simulink model "FWLowModel"  (R2020b)
settings: Solver=VariableStepAuto  StartTime=0.0  StopTime=inf  RelTol=1e-3
libraries: uavalgslib x1
settings Model: EnablePacing=on  Creator=ISR  LastModifiedBy=chenjiaqing

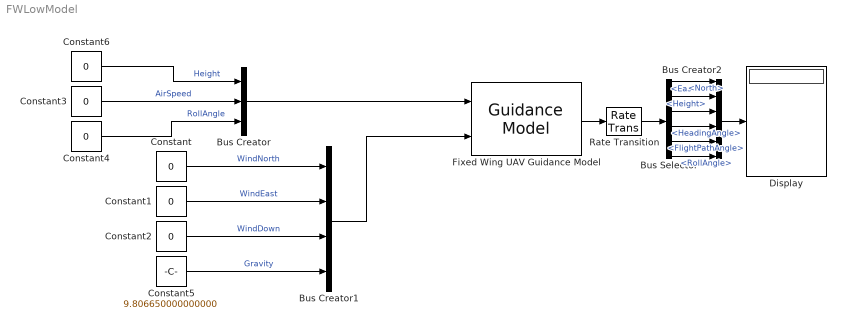
== system FWLowModel ==
  Bus Creator : BusCreator  Inputs=3  OutDataTypeStr=Bus: FixedWingControlBus  NonVirtualBus=on
  Bus Creator1 : BusCreator  Inputs=4  OutDataTypeStr=Bus: FixedWingEnvironmentBus  NonVirtualBus=on
  Bus Creator2 : BusCreator  Inputs=6
  Bus Selector : BusSelector  OutputSignals=North,East,Height,HeadingAngle,FlightPathAngle,RollAngle
  Constant{,1..4,6} (6 alike) : Constant  Value=0
  Constant5 : Constant  Value=9.806650000000000
  Display : Display
  Fixed Wing UAV Guidance Model : uavalgslib/Guidance Model  ModelType=FixedWingGuidance  SpecifiedDataType=double  SimulateUsing=Code generation  InitialWorldPositionMultirotor=[0; 0; 0]  InitialWorldVelocityMultirotor=[0; 0; 0]  InitialEulerZYXMultirotor=[0; 0; 0]  InitialBodyAngularRateRPYMultirotor=[0; 0; 0]  InitialThrustMultirotor=0  InitialNorthFixedWing=0  InitialEastFixedWing=0  InitialHeightFixedWing=0  InitialAirSpeedFixedWing=0  InitialHeadingAngleFixedWing=0  InitialFlightPathAngleFixedWing=0  InitialRollAngleFixedWing=0  InitialRollAngleRateFixedWing=0  PDRollMultirotor=[3402.97,116.67]  PDPitchMultirotor=[3402.97, 116.67]  PYawRateMultirotor=1950  PThrustMultirotor=3900  MassMultirotor=0.1  PHeightFixedWing=0.78  PHeadingAngleFixedWing=3.9  PFlightPathAngleFixedWing=3.9  PDRollFixedWing="[5.4448      4.6668]"  PAirSpeedFixedWing=7.8  FlightPathAngleLimitsFixedWing=[-pi/4, pi/4]  StateBusName='FixedWingStateBus'  ControlBusName='FixedWingControlBus'  EnvironmentBusName='FixedWingEnvironmentBus'  DataType=double
      settings: SourceProductName=UAV Toolbox
  Rate Transition : RateTransition  OutPortSampleTime=0.1
  wires:
  Fixed Wing UAV Guidance Model/1 -> Rate Transition/1
  Bus Selector/4 -> Bus Creator2/4  "<HeadingAngle>"
  Bus Creator2/1 -> Display/1
  Bus Selector/5 -> Bus Creator2/5  "<FlightPathAngle>"
  Bus Selector/6 -> Bus Creator2/6  "<RollAngle>"
  Bus Selector/2 -> Bus Creator2/2  "<East>"
  Bus Selector/3 -> Bus Creator2/3  "<Height>"
  Rate Transition/1 -> Bus Selector/1
  Constant3/1 -> Bus Creator/2  "AirSpeed"
  Constant4/1 -> Bus Creator/3  "RollAngle"
  Bus Selector/1 -> Bus Creator2/1  "<North>"
  Constant2/1 -> Bus Creator1/3  "WindDown"
  Bus Creator/1 -> Fixed Wing UAV Guidance Model/1
  Constant/1 -> Bus Creator1/1  "WindNorth"
  Constant1/1 -> Bus Creator1/2  "WindEast"
  Bus Creator1/1 -> Fixed Wing UAV Guidance Model/2
  Constant6/1 -> Bus Creator/1  "Height"
  Constant5/1 -> Bus Creator1/4  "Gravity"
